simulink model "enabled"  (R2020b)
settings: Solver=VariableStepAuto  StartTime=0.0  StopTime=1  MaxStep=0.01  RelTol=1e-3
settings Model: Creator=99003736  LastModifiedBy=99003736

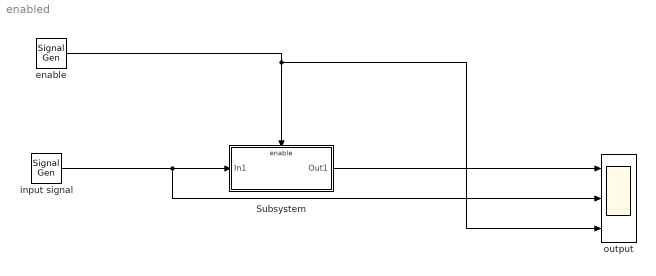
== system enabled ==
  Subsystem : Subsystem
  enable : SignalGenerator  WaveForm=square
  input signal : SignalGenerator  Frequency=3
  output : Scope  NumInputPorts=3
  wires:
  input signal/1 -> output/2, Subsystem/1(In1)
  Subsystem/1(Out1) -> output/1
  enable/1 -> output/3, Subsystem/Enable

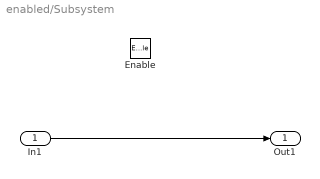
== system enabled/Subsystem ==
  In1 : Inport
  Enable : EnablePort  StatesWhenEnabling=reset
  Out1 : Outport
  wires:
  In1/1 -> Out1/1
